simulink model "xaui_simulator"  (Simulink 7.0)
settings: Solver=ode45  StartTime=0.0  StopTime=1000  RelTol=1e-3
undefined symbols (not defined in the file or in its folder): ROACH
libraries: xbsIndex_r4 x30, xps_library x14, casper_library x2, gavrt_library x1
settings Model: Creator=rprimian  LastModifiedBy=Administrator
settings OptimizationCC: InitFltsAndDblsToZero=off

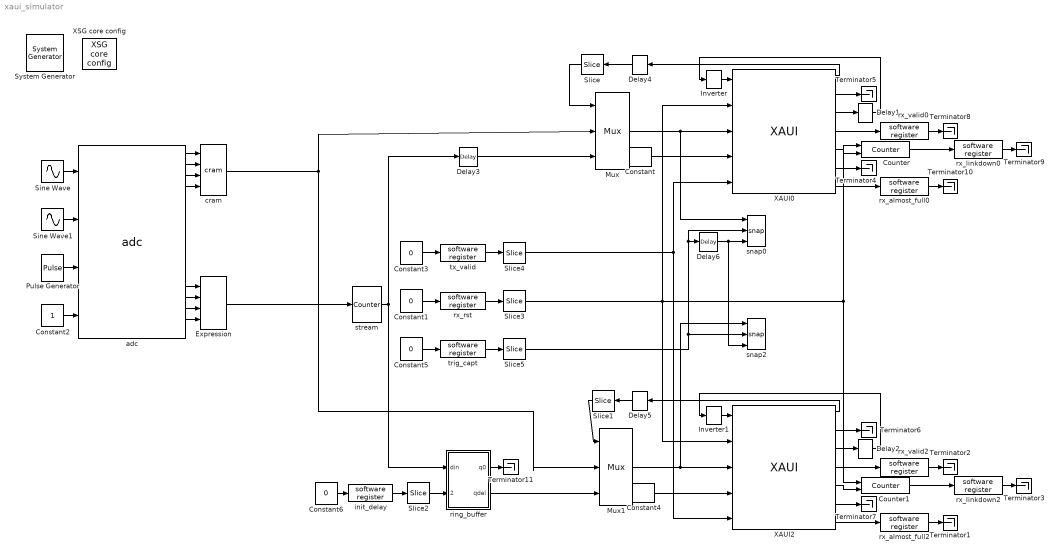
== system xaui_simulator ==
  " System Generator" : xbsIndex_r4/ System Generator  Tag=genX  SystemSampleTime=-1  xilinxfamily=virtex5  part=xc5vsx95t  speed=-1  package=ff1136  synthesis_tool=XST  clock_wrapper=Clock Enables  directory=./xaui_simulator/sysgen  testbench=off  simulink_period=1  sysclk_period=3.9063  dcm_input_clock_period=100  incr_netlist=off  trim_vbits=Everywhere in SubSystem  dbl_ovrd=According to Block Masks  core_generation=According to Block Masks  run_coregen=off  deprecated_control=off  eval_field=0  block_type=sysgen
      settings: block_version=11.3
  Constant : xbsIndex_r4/Constant  arith_type=Unsigned  const=0  n_bits=4  bin_pt=0  explicit_period=on  period=1  equ=P=C  opselect=C  inp2=PCIN>>17  opr=+  inp1=P  carry=CIN  dbl_ovrd=off  block_type=constant
      settings: block_version=11.3
  Constant{1,3,5..6} (4 alike) : Constant  Value=0  OutDataType=fixdt(1, 16)  OutScaling=2^0
  Constant2 : Constant  OutDataType=fixdt(1, 16)  OutScaling=2^0
  Constant4 : xbsIndex_r4/Constant  arith_type=Unsigned  const=0  n_bits=4  bin_pt=0  explicit_period=on  period=1  equ=P=C  opselect=C  inp2=PCIN>>17  opr=+  inp1=P  carry=CIN  dbl_ovrd=off  block_type=constant
      settings: block_version=11.3
  Counter : xbsIndex_r4/Counter  cnt_type=Free Running  cnt_to=Inf  operation=Up  start_count=0  cnt_by_val=1  arith_type=Unsigned  n_bits=32  bin_pt=0  load_pin=off  rst=on  en=on  explicit_period=on  period=1  dbl_ovrd=off  use_behavioral_HDL=off  use_rpm=off  implementation=Fabric  block_type=counter
      settings: block_version=11.3
  Counter1 : xbsIndex_r4/Counter  cnt_type=Free Running  cnt_to=Inf  operation=Up  start_count=0  cnt_by_val=1  arith_type=Unsigned  n_bits=32  bin_pt=0  load_pin=off  rst=on  en=on  explicit_period=on  period=1  dbl_ovrd=off  use_behavioral_HDL=off  use_rpm=off  implementation=Fabric  block_type=counter
      settings: block_version=11.3
  Delay1 : xbsIndex_r4/Delay  en=off  latency=32  dbl_ovrd=off  reg_retiming=off  block_type=delay
      settings: block_version=11.3
  Delay2 : xbsIndex_r4/Delay  en=off  latency=32  dbl_ovrd=off  reg_retiming=off  block_type=delay
      settings: block_version=11.3
  Delay3 : xbsIndex_r4/Delay  en=off  latency=8  dbl_ovrd=off  reg_retiming=on  block_type=delay
  Delay4 : xbsIndex_r4/Delay  Orientation=left  en=off  latency=20  dbl_ovrd=off  reg_retiming=off  block_type=delay
      settings: block_version=11.3
  Delay5 : xbsIndex_r4/Delay  Orientation=left  en=off  latency=20  dbl_ovrd=off  reg_retiming=off  block_type=delay
      settings: block_version=11.3
  Delay6 : xbsIndex_r4/Delay  en=off  latency=8  dbl_ovrd=off  reg_retiming=on  block_type=delay
  Expression : xbsIndex_r4/Expression  expression=a | b | c | d  align_bp=on  en=off  latency=0  precision=Full  arith_type=Unsigned  n_bits=16  bin_pt=0  dbl_ovrd=off  block_type=expr
      settings: block_version=11.3
  Inverter : xbsIndex_r4/Inverter  en=off  latency=0  dbl_ovrd=off  block_type=inv
      settings: block_version=11.3
  Inverter1 : xbsIndex_r4/Inverter  en=off  latency=0  dbl_ovrd=off  block_type=inv
      settings: block_version=11.3
  Mux : xbsIndex_r4/Mux  inputs=2  en=off  latency=0  precision=Full  arith_type=Unsigned  n_bits=16  bin_pt=14  quantization=Truncate  overflow=Wrap  dbl_ovrd=off  block_type=mux
      settings: block_version=11.3
  Mux1 : xbsIndex_r4/Mux  inputs=2  en=off  latency=0  precision=Full  arith_type=Unsigned  n_bits=16  bin_pt=14  quantization=Truncate  overflow=Wrap  dbl_ovrd=off  block_type=mux
      settings: block_version=11.3
  Pulse Generator : DiscretePulseGenerator  Period=1000  SampleTime=0.25
  Sine Wave : Sin  SineType=Sample based  Amplitude=0.25  SampleTime=0.25
  Sine Wave1 : Sin  SineType=Sample based  Amplitude=0.25  SampleTime=0.25
  Slice : xbsIndex_r4/Slice  Orientation=left  nbits=1  boolean_output=on  mode=Lower Bit Location + Width  bit1=0  base1=MSB of Input  bit0=0  base0=LSB of Input  dbl_ovrd=off  block_type=slice
      settings: block_version=11.3
  Slice1 : xbsIndex_r4/Slice  Orientation=left  nbits=1  boolean_output=on  mode=Lower Bit Location + Width  bit1=0  base1=MSB of Input  bit0=0  base0=LSB of Input  dbl_ovrd=off  block_type=slice
      settings: block_version=11.3
  Slice2 : xbsIndex_r4/Slice  nbits=4  boolean_output=off  mode=Lower Bit Location + Width  bit1=0  base1=MSB of Input  bit0=0  base0=LSB of Input  dbl_ovrd=off  block_type=slice
      settings: block_version=11.3
  Slice3 : xbsIndex_r4/Slice  nbits=1  boolean_output=on  mode=Lower Bit Location + Width  bit1=0  base1=MSB of Input  bit0=0  base0=LSB of Input  dbl_ovrd=off  block_type=slice
      settings: block_version=11.3
  Slice4 : xbsIndex_r4/Slice  nbits=1  boolean_output=on  mode=Lower Bit Location + Width  bit1=0  base1=MSB of Input  bit0=0  base0=LSB of Input  dbl_ovrd=off  block_type=slice
      settings: block_version=11.3
  Slice5 : xbsIndex_r4/Slice  nbits=1  boolean_output=on  mode=Lower Bit Location + Width  bit1=0  base1=MSB of Input  bit0=0  base0=LSB of Input  dbl_ovrd=off  block_type=slice
      settings: block_version=11.3
  Terminator{1..11} (11 alike) : Terminator
  XAUI0 : xps_library/XAUI  Tag=xps:xaui  SystemSampleTime=-1  demux=2  port=ROACH:0  open_phy=off  show_param=off  pre_emph=3  swing=800
      link override convert_tx_data: n_bits=32
      link override convert_tx_outofband: n_bits=4
      link override xaui_simulator_XAUI0_rx_data: n_bits=32
      link override xaui_simulator_XAUI0_rx_outofband: n_bits=4
  XAUI2 : xps_library/XAUI  Tag=xps:xaui  SystemSampleTime=-1  demux=2  port=ROACH:2  open_phy=off  show_param=off  pre_emph=3  swing=800
      link override convert_tx_data: n_bits=32
      link override convert_tx_outofband: n_bits=4
      link override xaui_simulator_XAUI2_rx_data: n_bits=32
      link override xaui_simulator_XAUI2_rx_outofband: n_bits=4
  XSG core config : xps_library/XSG core config  Tag=xps:xsg  SystemSampleTime=-1  hw_sys=ROACH:sx95t  ibob_linux=off  clk_src=adc0_clk  iBOB_clk_src=sys_clk  BEE2_ctrl_clk_src=sys_clk  BEE2_usr_clk_src=sys_clk  ROACH_clk_src=adc0_clk  CORR_clk_src=sys_clk  gpio_clk_io_group=iBOB:sma  gpio_clk_bit_index=0  clk_rate=256  sample_period=1  synthesis_tool=XST  mpc_type=powerpc440_ext
  adc : xps_library/adc  Tag=xps:adc  SystemSampleTime=-1  adc_brd=adc0  adc_clk_rate=1024  adc_interleave=off  sample_period=1
  cram : gavrt_library/cram  SystemSampleTime=-1  num_slice=4
  init_delay : xps_library/software register  Tag=xps:sw_reg  SystemSampleTime=-1  io_dir=From Processor  arith_type=Unsigned  bitwidth=32  bin_pt=0  sample_period=1  gw_name=xaui_simulator_init_delay_user_data_out
      link override xaui_simulator_init_delay_user_data_out: arith_type=Unsigned  n_bits=32  bin_pt=0  period=1
  ring_buffer : Subsystem
  rx_almost_full0 : xps_library/software register  Tag=xps:sw_reg  SystemSampleTime=-1  io_dir=To Processor  arith_type=Unsigned  bitwidth=32  bin_pt=0  sample_period=1  gw_name=xaui_simulator_rx_almost_full0_user_data_in
      link override convert: arith_type=Unsigned  n_bits=32  bin_pt=0
  rx_almost_full2 : xps_library/software register  Tag=xps:sw_reg  SystemSampleTime=-1  io_dir=To Processor  arith_type=Unsigned  bitwidth=32  bin_pt=0  sample_period=1  gw_name=xaui_simulator_rx_almost_full2_user_data_in
      link override convert: arith_type=Unsigned  n_bits=32  bin_pt=0
  rx_linkdown0 : xps_library/software register  Tag=xps:sw_reg  SystemSampleTime=-1  io_dir=To Processor  arith_type=Unsigned  bitwidth=32  bin_pt=0  sample_period=1  gw_name=xaui_simulator_rx_linkdown0_user_data_in
      link override convert: arith_type=Unsigned  n_bits=32  bin_pt=0
  rx_linkdown2 : xps_library/software register  Tag=xps:sw_reg  SystemSampleTime=-1  io_dir=To Processor  arith_type=Unsigned  bitwidth=32  bin_pt=0  sample_period=1  gw_name=xaui_simulator_rx_linkdown2_user_data_in
      link override convert: arith_type=Unsigned  n_bits=32  bin_pt=0
  rx_rst : xps_library/software register  Tag=xps:sw_reg  SystemSampleTime=-1  io_dir=From Processor  arith_type=Unsigned  bitwidth=32  bin_pt=0  sample_period=1  gw_name=xaui_simulator_rx_rst_user_data_out
      link override xaui_simulator_rx_rst_user_data_out: arith_type=Unsigned  n_bits=32  bin_pt=0  period=1
  rx_valid0 : xps_library/software register  Tag=xps:sw_reg  SystemSampleTime=-1  io_dir=To Processor  arith_type=Unsigned  bitwidth=32  bin_pt=0  sample_period=1  gw_name=xaui_simulator_rx_valid0_user_data_in
      link override convert: arith_type=Unsigned  n_bits=32  bin_pt=0
  rx_valid2 : xps_library/software register  Tag=xps:sw_reg  SystemSampleTime=-1  io_dir=To Processor  arith_type=Unsigned  bitwidth=32  bin_pt=0  sample_period=1  gw_name=xaui_simulator_rx_valid2_user_data_in
      link override convert: arith_type=Unsigned  n_bits=32  bin_pt=0
  snap0 : casper_library/Scopes/snap  SystemSampleTime=-1  nsamples=11
      link override addr/convert: arith_type=Unsigned  n_bits=32  bin_pt=0
      link override bram/convert_din: arith_type=Unsigned
      link override bram/mem/sim_data_in: arith_type=Unsigned
      link override bram/xaui_simulator_snap0_bram_data_out: arith_type=Unsigned
      link override ctrl/xaui_simulator_snap0_ctrl_user_data_out: arith_type=Unsigned  n_bits=32  bin_pt=0  period=1
  snap2 : casper_library/Scopes/snap  SystemSampleTime=-1  nsamples=11
      link override addr/convert: arith_type=Unsigned  n_bits=32  bin_pt=0
      link override bram/convert_din: arith_type=Unsigned
      link override bram/mem/sim_data_in: arith_type=Unsigned
      link override bram/xaui_simulator_snap2_bram_data_out: arith_type=Unsigned
      link override ctrl/xaui_simulator_snap2_ctrl_user_data_out: arith_type=Unsigned  n_bits=32  bin_pt=0  period=1
  stream : xbsIndex_r4/Counter  cnt_type=Free Running  cnt_to=Inf  operation=Up  start_count=0  cnt_by_val=1  arith_type=Unsigned  n_bits=32  bin_pt=0  load_pin=off  rst=on  en=off  explicit_period=on  period=1  dbl_ovrd=off  use_behavioral_HDL=off  use_rpm=off  implementation=Fabric  block_type=counter
  trig_capt : xps_library/software register  Tag=xps:sw_reg  SystemSampleTime=-1  io_dir=From Processor  arith_type=Unsigned  bitwidth=32  bin_pt=0  sample_period=1  gw_name=xaui_simulator_trig_capt_user_data_out
      link override xaui_simulator_trig_capt_user_data_out: arith_type=Unsigned  n_bits=32  bin_pt=0  period=1
  tx_valid : xps_library/software register  Tag=xps:sw_reg  SystemSampleTime=-1  io_dir=From Processor  arith_type=Unsigned  bitwidth=32  bin_pt=0  sample_period=1  gw_name=xaui_simulator_tx_valid_user_data_out
      link override xaui_simulator_tx_valid_user_data_out: arith_type=Unsigned  n_bits=32  bin_pt=0  period=1
  wires:
  stream/1 -> Delay3/1, ring_buffer/1(din)
  init_delay/1 -> Slice2/1
  Constant6/1 -> init_delay/1
  Mux/1 -> XAUI0/3, snap0/1
  Mux1/1 -> XAUI2/3, snap2/1
  XAUI0/1 -> Delay4/1
  Slice1/1 -> Mux1/1
  Delay1/1 -> Inverter/1
  Inverter/1 -> XAUI0/1
  XAUI0/3 -> Delay1/1
  Delay2/1 -> Inverter1/1
  Inverter1/1 -> XAUI2/1
  XAUI2/3 -> Delay2/1
  XAUI2/1 -> Delay5/1
  Constant/1 -> XAUI0/4
  Slice2/1 -> ring_buffer/2(delay)
  rx_rst/1 -> Slice3/1
  Constant1/1 -> rx_rst/1
  Delay3/1 -> Mux/3
  ring_buffer/2(qdel) -> Mux1/3
  XAUI0/4 -> rx_valid0/1
  rx_valid0/1 -> Terminator8/1
  rx_linkdown0/1 -> Terminator9/1
  rx_almost_full0/1 -> Terminator10/1
  XAUI0/7 -> rx_almost_full0/1
  XAUI2/4 -> rx_valid2/1
  rx_valid2/1 -> Terminator2/1
  rx_linkdown2/1 -> Terminator3/1
  rx_almost_full2/1 -> Terminator1/1
  XAUI2/7 -> rx_almost_full2/1
  XAUI0/6 -> Terminator4/1
  XAUI0/2 -> Terminator5/1
  XAUI2/2 -> Terminator6/1
  XAUI2/6 -> Terminator7/1
  ring_buffer/1(q0) -> Terminator11/1
  Constant4/1 -> XAUI2/4
  Slice3/1 -> XAUI0/2, XAUI2/2, Counter/1, Counter1/1
  Sine Wave/1 -> adc/1
  Sine Wave1/1 -> adc/2
  Pulse Generator/1 -> adc/3
  Constant2/1 -> adc/4
  adc/13 -> Expression/1
  adc/14 -> Expression/2
  adc/15 -> Expression/3
  adc/16 -> Expression/4
  Expression/1 -> stream/1
  adc/1 -> cram/1
  adc/2 -> cram/2
  adc/3 -> cram/3
  adc/4 -> cram/4
  cram/1 -> Mux/2, Mux1/2
  Delay4/1 -> Slice/1
  Delay5/1 -> Slice1/1
  Constant3/1 -> tx_valid/1
  tx_valid/1 -> Slice4/1
  Slice4/1 -> XAUI0/5, XAUI2/5
  Constant5/1 -> trig_capt/1
  trig_capt/1 -> Slice5/1
  Slice5/1 -> snap2/2, snap0/2, Delay6/1
  Delay6/1 -> snap0/3, snap2/3
  Counter/1 -> rx_linkdown0/1
  Counter1/1 -> rx_linkdown2/1
  XAUI0/5 -> Counter/2
  XAUI2/5 -> Counter1/2
  Slice/1 -> Mux/1

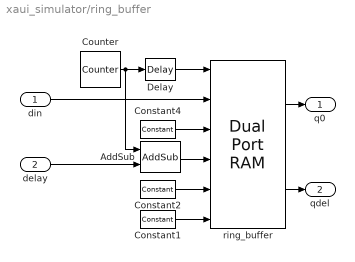
== system xaui_simulator/ring_buffer ==
  din : Inport
  delay : Inport  Port=2
  AddSub : xbsIndex_r4/AddSub  mode=Subtraction  use_carryin=off  use_carryout=off  en=off  latency=2  precision=User Defined  arith_type=Unsigned  n_bits=4  bin_pt=0  quantization=Truncate  overflow=Wrap  dbl_ovrd=off  use_behavioral_HDL=off  pipelined=off  use_rpm=on  hw_selection=Fabric  block_type=addsub
      settings: block_version=11.3
  Constant1 : xbsIndex_r4/Constant  arith_type=Boolean  const=0  n_bits=4  bin_pt=0  explicit_period=on  period=1  equ=P=C  opselect=C  inp2=PCIN>>17  opr=+  inp1=P  carry=CIN  dbl_ovrd=off  block_type=constant
      settings: block_version=11.3
  Constant2 : xbsIndex_r4/Constant  arith_type=Unsigned  const=0  n_bits=32  bin_pt=0  explicit_period=on  period=1  equ=P=C  opselect=C  inp2=PCIN>>17  opr=+  inp1=P  carry=CIN  dbl_ovrd=off  block_type=constant
      settings: block_version=11.3
  Constant4 : xbsIndex_r4/Constant  arith_type=Boolean  const=1  n_bits=4  bin_pt=0  explicit_period=on  period=1  equ=P=C  opselect=C  inp2=PCIN>>17  opr=+  inp1=P  carry=CIN  dbl_ovrd=off  block_type=constant
      settings: block_version=11.3
  Counter : xbsIndex_r4/Counter  cnt_type=Free Running  cnt_to=Inf  operation=Up  start_count=0  cnt_by_val=1  arith_type=Unsigned  n_bits=4  bin_pt=0  load_pin=off  rst=off  en=off  explicit_period=on  period=1  dbl_ovrd=off  use_behavioral_HDL=off  use_rpm=off  implementation=Fabric  block_type=counter
      settings: block_version=11.3
  Delay : xbsIndex_r4/Delay  en=off  latency=2  dbl_ovrd=off  reg_retiming=off  block_type=delay
      settings: block_version=11.3
  ring_buffer : xbsIndex_r4/Dual Port RAM  depth=16  initVector=zeros(1,16)  distributed_mem=Block RAM  init_a=0  init_b=0  rst_a=off  rst_b=off  en_a=off  en_b=off  latency=2  write_mode_A=Read After Write  write_mode_B=Read After Write  dbl_ovrd=off  optimize=Speed  use_rpm=off  block_type=dpram
      settings: block_version=11.3
  q0 : Outport
  qdel : Outport  Port=2
  wires:
  Counter/1 -> AddSub/1, Delay/1
  AddSub/1 -> ring_buffer/4
  Constant4/1 -> ring_buffer/3
  din/1 -> ring_buffer/2
  ring_buffer/1 -> q0/1
  delay/1 -> AddSub/2
  ring_buffer/2 -> qdel/1
  Delay/1 -> ring_buffer/1
  Constant1/1 -> ring_buffer/6
  Constant2/1 -> ring_buffer/5
